simulink library "halout"  (R2021b)
settings: Solver=VariableStepAuto  StartTime=0.0  StopTime=10.0  RelTol=1e-3
undefined symbols (not defined in the file): C_TASK_5MS_S, KHAL_CAN1TxReq_flg, KHAL_CAN2TxReq_flg, KHAL_CAN3TxReq_flg, KHAL_CAN4TxReq_flg, KHAL_CAN5TxReq_flg, KHAL_CAN6TxReq_flg, KHAL_CAN7TxReq_flg, TRUE
libraries: FVT_lib x65, simulink x6
(part 1 of 6)
settings Model: Creator=13168  LastModifiedBy=FVT22063
settings SolverCC: AlgebraicLoopSolver=TrustRegion
settings DataIOCC: SaveFormat=Array  SignalLoggingSaveFormat=ModelDataLogs  ReturnWorkspaceOutputs=off
settings OptimizationCC: BlockReduction=off  BooleanDataType=off
settings DebuggingCC: SaveWithParameterizedLinksMsg=none  UnderspecifiedInitializationDetection=Classic  MergeDetectMultiDrivingBlocksExec=none  SignalResolutionControl=TryResolveAllWithWarning  SFMachineParentedDataDiag=warning
settings HardwareCC: TargetUnknown=on
settings ModelReferenceCC: PropagateSignalLabelsOutOfModel=off
settings ConfigComp: CovMetricSettings=dw  CovSaveCumulativeToWorkspaceVar=on  CovSaveSingleToWorkspaceVar=on

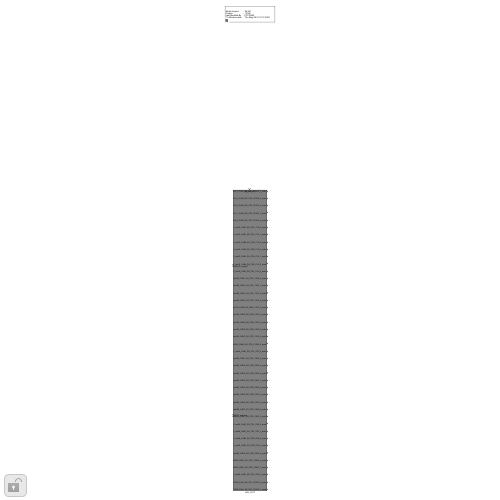
[thumbnail: Simulink's stored preview of the top-level diagram]
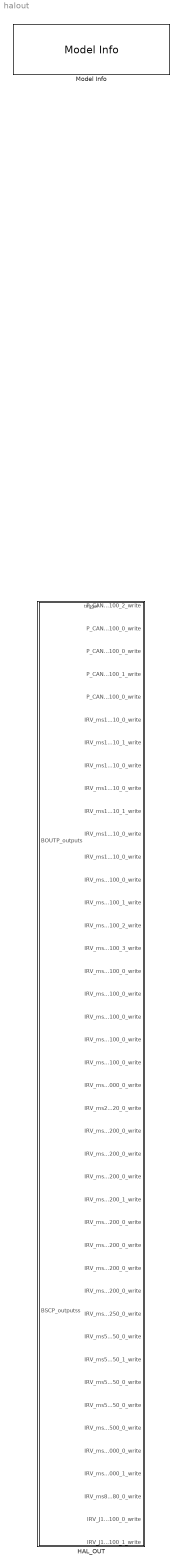
== system halout ==
  HAL_OUT : Subsystem
      settings: RTWSystemCode=Nonreusable function  RTWFcnNameOpts=Use subsystem name  RTWFileNameOpts=Use subsystem name
  Model Info : simulink/Model-Wide Utilities/Model Info  Frame=on  DisplayStringWithTags=|  HorizontalTextAlignment=Left  LeftAlignmentValue=0.02
      | Model Version        : %<ModelVersion>
      | Creator                   : %<Creator>
      | Last Modified By    : %<LastModifiedBy>
      | Modification date    : %<LastModificationDate>

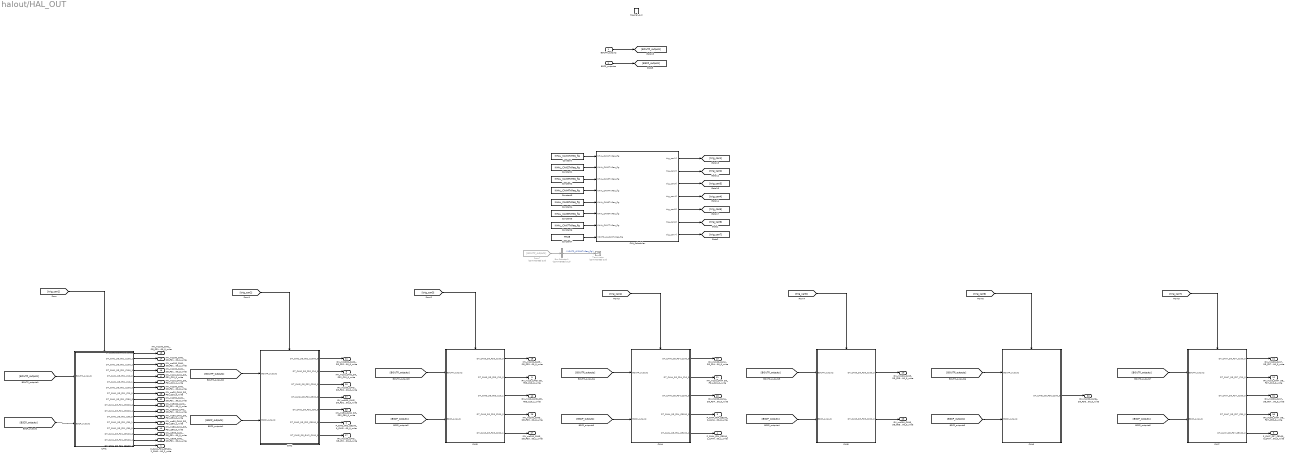
== system halout/HAL_OUT ==
  BOUTP_outputs : Inport  OutDataTypeStr=Bus: BOUTP_outputs
  BSCP_outputss : Inport  Port=2  OutDataTypeStr=Bus: BSCP_outputs
  trig_hal_out : TriggerPort  TriggerType=function-call  VariantControl=(inherit)
  Bus Selector1 : BusSelector  Commented=on  OutputSignals=VOUTP_AllCANTxReq_flg
  CAN1 : Subsystem  TreatAsAtomicUnit=on
  CAN2 : Subsystem  TreatAsAtomicUnit=on
  CAN3 : Subsystem  TreatAsAtomicUnit=on
  CAN4 : Subsystem  TreatAsAtomicUnit=on
  CAN5 : Subsystem  TreatAsAtomicUnit=on
  CAN6 : Subsystem  TreatAsAtomicUnit=on
  CAN7 : Subsystem  TreatAsAtomicUnit=on
  CAN_Scheduler : Stateflow chart  TreatAsAtomicUnit=on
  Constant : Constant  Value=KHAL_CAN1TxReq_flg
  Constant1 : Constant  Value=KHAL_CAN2TxReq_flg
  Constant2 : Constant  Value=KHAL_CAN3TxReq_flg
  Constant3 : Constant  Value=KHAL_CAN4TxReq_flg
  Constant4 : Constant  Value=KHAL_CAN5TxReq_flg
  Constant5 : Constant  Value=KHAL_CAN6TxReq_flg
  Constant6 : Constant  Value=KHAL_CAN7TxReq_flg
  Constant7 : Constant  Value=TRUE
  From7 : From  Commented=on  GotoTag=BOUTP_outputs
  Terminator : Terminator  Commented=on
  P_CAN1_FD1_CE100_2_CAN1_SG_FD1_CE100_2_write : Outport  OutDataTypeStr=Bus: DT_CAN1_SG_FD1_CE100_2
  P_CAN2_FD2_CE100_0_CAN2_SG_FD2_CE100_0_write : Outport  Port=2  OutDataTypeStr=Bus: DT_CAN2_SG_FD2_CE100_0
  P_CAN4_FD4_CE100_0_CAN4_SG_FD4_CE100_0_write : Outport  Port=3  OutDataTypeStr=Bus: DT_CAN4_SG_FD4_CE100_0
  P_CAN4_FD4_CE100_1_CAN4_SG_FD4_CE100_1_write : Outport  Port=4  OutDataTypeStr=Bus: DT_CAN4_SG_FD4_CE100_1
  P_CAN7_FD7_CE100_0_CAN7_SG_FD7_CE100_0_write : Outport  Port=5  OutDataTypeStr=Bus: DT_CAN7_SG_FD7_CE100_0
  IRV_ms10_CAN1_SG_FD1_C10_0_write : Outport  Port=6  OutDataTypeStr=Bus: DT_CAN1_SG_FD1_C10_0
  IRV_ms10_CAN1_SG_FD1_C10_1_write : Outport  Port=7  OutDataTypeStr=Bus: DT_CAN1_SG_FD1_C10_1
  IRV_ms10_CAN2_SG_FD2_C10_0_write : Outport  Port=8  OutDataTypeStr=Bus: DT_CAN2_SG_FD2_C10_0
  IRV_ms10_CAN3_SG_FD3_C10_0_write : Outport  Port=9  OutDataTypeStr=Bus: DT_CAN3_SG_FD3_C10_0
  IRV_ms10_CAN3_SG_FD3_C10_1_write : Outport  Port=10  OutDataTypeStr=Bus: DT_CAN3_SG_FD3_C10_1
  IRV_ms10_CAN4_SG_FD4_C10_0_write : Outport  Port=11  OutDataTypeStr=Bus: DT_CAN4_SG_FD4_C10_0
  IRV_ms10_CAN7_SG_FD7_C10_0_write : Outport  Port=12  OutDataTypeStr=Bus: DT_CAN7_SG_FD7_C10_0
  IRV_ms100_CAN1_SG_FD1_C100_0_write : Outport  Port=13  OutDataTypeStr=Bus: DT_CAN1_SG_FD1_C100_0
  IRV_ms100_CAN1_SG_FD1_C100_1_write : Outport  Port=14  OutDataTypeStr=Bus: DT_CAN1_SG_FD1_C100_1
  IRV_ms100_CAN1_SG_FD1_C100_2_write : Outport  Port=15  OutDataTypeStr=Bus: DT_CAN1_SG_FD1_C100_2
  IRV_ms100_CAN1_SG_FD1_C100_3_write : Outport  Port=16  OutDataTypeStr=Bus: DT_CAN1_SG_FD1_C100_3
  IRV_ms100_CAN2_SG_GW2_C100_0_write : Outport  Port=17  OutDataTypeStr=Bus: DT_CAN2_SG_GW2_C100_0
  IRV_ms100_CAN3_SG_FD3_C100_0_write : Outport  Port=18  OutDataTypeStr=Bus: DT_CAN3_SG_FD3_C100_0
  IRV_ms100_CAN4_SG_FD4_C100_0_write : Outport  Port=19  OutDataTypeStr=Bus: DT_CAN4_SG_FD4_C100_0
  IRV_ms100_CAN5_SG_FD5_C100_0_write : Outport  Port=20  OutDataTypeStr=Bus: DT_CAN5_SG_FD5_C100_0
  IRV_ms100_CAN7_SG_FD7_C100_0_write : Outport  Port=21  OutDataTypeStr=Bus: DT_CAN7_SG_FD7_C100_0
  IRV_ms1000_CAN2_SG_FD2_C1000_0_write : Outport  Port=22  OutDataTypeStr=Bus: DT_CAN2_SG_FD2_C1000_0
  IRV_ms20_CAN1_SG_FD1_C20_0_write : Outport  Port=23  OutDataTypeStr=Bus: DT_CAN1_SG_FD1_C20_0
  IRV_ms200_CAN1_SG_FD1_C200_0_write : Outport  Port=24  OutDataTypeStr=Bus: DT_CAN1_SG_FD1_C200_0
  IRV_ms200_CAN2_SG_FD2_C200_0_write : Outport  Port=25  OutDataTypeStr=Bus: DT_CAN2_SG_FD2_C200_0
  IRV_ms200_CAN3_SG_FD3_C200_0_write : Outport  Port=26  OutDataTypeStr=Bus: DT_CAN3_SG_FD3_C200_0
  IRV_ms200_CAN3_SG_FD3_C200_1_write : Outport  Port=27  OutDataTypeStr=Bus: DT_CAN3_SG_FD3_C200_1
  IRV_ms200_CAN4_SG_FD4_C200_0_write : Outport  Port=28  OutDataTypeStr=Bus: DT_CAN4_SG_FD4_C200_0
  IRV_ms200_CAN5_SG_FD5_C200_0_write : Outport  Port=29  OutDataTypeStr=Bus: DT_CAN5_SG_FD5_C200_0
  IRV_ms200_CAN6_SG_FD6_C200_0_write : Outport  Port=30  OutDataTypeStr=Bus: DT_CAN6_SG_FD6_C200_0
  IRV_ms200_CAN7_SG_FD7_C200_0_write : Outport  Port=31  OutDataTypeStr=Bus: DT_CAN7_SG_FD7_C200_0
  IRV_ms250_CAN1_SG_FD1_C250_0_write : Outport  Port=32  OutDataTypeStr=Bus: DT_CAN1_SG_FD1_C250_0
  IRV_ms50_CAN1_SG_FD1_C50_0_write : Outport  Port=33  OutDataTypeStr=Bus: DT_CAN1_SG_FD1_C50_0
  IRV_ms50_CAN1_SG_FD1_C50_1_write : Outport  Port=34  OutDataTypeStr=Bus: DT_CAN1_SG_FD1_C50_1
  IRV_ms50_CAN2_SG_FD2_C50_0_write : Outport  Port=35  OutDataTypeStr=Bus: DT_CAN2_SG_FD2_C50_0
  IRV_ms50_CAN7_SG_FD7_C50_0_write : Outport  Port=36  OutDataTypeStr=Bus: DT_CAN7_SG_FD7_C50_0
  IRV_ms500_CAN2_SG_FD2_C500_0_write : Outport  Port=37  OutDataTypeStr=Bus: DT_CAN2_SG_FD2_C500_0
  IRV_ms5000_CAN1_SG_FD1_C5000_0_write : Outport  Port=38  OutDataTypeStr=Bus: DT_CAN1_SG_FD1_C5000_0
  IRV_ms5000_CAN1_SG_FD1_C5000_1_write : Outport  Port=39  OutDataTypeStr=Bus: DT_CAN1_SG_FD1_C5000_1
  IRV_ms80_CAN1_SG_FD1_C80_0_write : Outport  Port=40  OutDataTypeStr=Bus: DT_CAN1_SG_FD1_C80_0
  IRV_J1939_CAN1_SG_FD1_CE100_0_write : Outport  Port=41  OutDataTypeStr=Bus: DT_CAN1_SG_FD1_CE100_0
  IRV_J1939_CAN1_SG_FD1_CE100_1_write : Outport  Port=42  OutDataTypeStr=Bus: DT_CAN1_SG_FD1_CE100_1
  wires:
  BSCP_outputss/1 -> [BSCP_outputs]
  BOUTP_outputs/1 -> [BOUTP_outputs]
  Constant1/1 -> CAN_Scheduler/2(KHAL_CAN2TxReq_flg)
  Constant3/1 -> CAN_Scheduler/4(KHAL_CAN4TxReq_flg)
  CAN_Scheduler/1(trig_can1()) -> [trig_can1]
  CAN_Scheduler/2(trig_can2()) -> [trig_can2]
  Constant/1 -> CAN_Scheduler/1(KHAL_CAN1TxReq_flg)
  CAN_Scheduler/4(trig_can4()) -> [trig_can4]
  CAN_Scheduler/5(trig_can5()) -> [trig_can5]
  Constant4/1 -> CAN_Scheduler/5(KHAL_CAN5TxReq_flg)
  Constant2/1 -> CAN_Scheduler/3(KHAL_CAN3TxReq_flg)
  CAN_Scheduler/3(trig_can3()) -> [trig_can3]
  [trig_can1] -> CAN1/Trigger
  [trig_can4] -> CAN4/Trigger
  [trig_can5] -> CAN5/Trigger
  [trig_can2] -> CAN2/Trigger
  Constant5/1 -> CAN_Scheduler/6(KHAL_CAN6TxReq_flg)
  CAN_Scheduler/6(trig_can6()) -> [trig_can6]
  [trig_can6] -> CAN6/Trigger
  [trig_can3] -> CAN3/Trigger
  CAN_Scheduler/7(trig_can7()) -> [trig_can7]
  Constant6/1 -> CAN_Scheduler/7(KHAL_CAN7TxReq_flg)
  [trig_can7] -> CAN7/Trigger
  From7/1 -> Bus Selector1/1
  Bus Selector1/1 -> Terminator/1  "<VOUTP_AllCANTxReq_flg>"
  Constant7/1 -> CAN_Scheduler/8(VOUTP_ALLCANTxReq_flg)
  CAN1/1(DT_CAN1_SG_FD1_C100_0) -> IRV_ms100_CAN1_SG_FD1_C100_0_write/1
  CAN2/2(DT_CAN2_SG_FD2_C10_0) -> IRV_ms10_CAN2_SG_FD2_C10_0_write/1
  CAN7/5(DT_CAN7_SG_FD7_CE100_0) -> P_CAN7_FD7_CE100_0_CAN7_SG_FD7_CE100_0_write/1
  CAN1/2(DT_CAN1_SG_FD1_C100_1) -> IRV_ms100_CAN1_SG_FD1_C100_1_write/1
  [BSCP_outputs] -> CAN2/2(BSCP_outputs)
  [BOUTP_outputs] -> CAN2/1(BOUTP_outputs)
  CAN1/17(DT_CAN1_SG_FD1_CE100_2) -> P_CAN1_FD1_CE100_2_CAN1_SG_FD1_CE100_2_write/1
  [BSCP_outputs] -> CAN1/2(BSCP_outputs)
  CAN7/2(DT_CAN7_SG_FD7_C10_0) -> IRV_ms10_CAN7_SG_FD7_C10_0_write/1
  CAN1/16(DT_CAN1_SG_FD1_CE100_1) -> IRV_J1939_CAN1_SG_FD1_CE100_1_write/1
  CAN2/6(DT_CAN2_SG_FD2_CE100_0) -> P_CAN2_FD2_CE100_0_CAN2_SG_FD2_CE100_0_write/1
  CAN1/15(DT_CAN1_SG_FD1_CE100_0) -> IRV_J1939_CAN1_SG_FD1_CE100_0_write/1
  CAN1/6(DT_CAN1_SG_FD1_C10_1) -> IRV_ms10_CAN1_SG_FD1_C10_1_write/1
  CAN1/14(DT_CAN1_SG_FD1_C80_0) -> IRV_ms80_CAN1_SG_FD1_C80_0_write/1
  CAN1/5(DT_CAN1_SG_FD1_C10_0) -> IRV_ms10_CAN1_SG_FD1_C10_0_write/1
  CAN1/11(DT_CAN1_SG_FD1_C5000_1) -> IRV_ms5000_CAN1_SG_FD1_C5000_1_write/1
  CAN1/10(DT_CAN1_SG_FD1_C5000_0) -> IRV_ms5000_CAN1_SG_FD1_C5000_0_write/1
  CAN2/4(DT_CAN2_SG_FD2_C500_0) -> IRV_ms500_CAN2_SG_FD2_C500_0_write/1
  CAN7/4(DT_CAN7_SG_FD7_C50_0) -> IRV_ms50_CAN7_SG_FD7_C50_0_write/1
  CAN2/5(DT_CAN2_SG_FD2_C50_0) -> IRV_ms50_CAN2_SG_FD2_C50_0_write/1
  CAN1/9(DT_CAN1_SG_FD1_C250_0) -> IRV_ms250_CAN1_SG_FD1_C250_0_write/1
  CAN6/1(DT_CAN6_SG_FD6_C200_0) -> IRV_ms200_CAN6_SG_FD6_C200_0_write/1
  CAN5/2(DT_CAN5_SG_FD5_C200_0) -> IRV_ms200_CAN5_SG_FD5_C200_0_write/1
  CAN4/3(DT_CAN4_SG_FD4_C200_0) -> IRV_ms200_CAN4_SG_FD4_C200_0_write/1
  CAN3/5(DT_CAN3_SG_FD3_C200_1) -> IRV_ms200_CAN3_SG_FD3_C200_1_write/1
  CAN2/3(DT_CAN2_SG_FD2_C200_0) -> IRV_ms200_CAN2_SG_FD2_C200_0_write/1
  CAN1/7(DT_CAN1_SG_FD1_C200_0) -> IRV_ms200_CAN1_SG_FD1_C200_0_write/1
  CAN3/4(DT_CAN3_SG_FD3_C200_0) -> IRV_ms200_CAN3_SG_FD3_C200_0_write/1
  CAN1/8(DT_CAN1_SG_FD1_C20_0) -> IRV_ms20_CAN1_SG_FD1_C20_0_write/1
  CAN3/3(DT_CAN3_SG_FD3_C10_1) -> IRV_ms10_CAN3_SG_FD3_C10_1_write/1
  CAN2/1(DT_CAN2_SG_FD2_C1000_0) -> IRV_ms1000_CAN2_SG_FD2_C1000_0_write/1
  CAN4/4(DT_CAN4_SG_FD4_CE100_0) -> P_CAN4_FD4_CE100_0_CAN4_SG_FD4_CE100_0_write/1
  CAN3/2(DT_CAN3_SG_FD3_C10_0) -> IRV_ms10_CAN3_SG_FD3_C10_0_write/1
  CAN7/1(DT_CAN7_SG_FD7_C100_0) -> IRV_ms100_CAN7_SG_FD7_C100_0_write/1
  CAN1/12(DT_CAN1_SG_FD1_C50_0) -> IRV_ms50_CAN1_SG_FD1_C50_0_write/1
  CAN5/1(DT_CAN5_SG_FD5_C100_0) -> IRV_ms100_CAN5_SG_FD5_C100_0_write/1
  CAN4/1(DT_CAN4_SG_FD4_C100_0) -> IRV_ms100_CAN4_SG_FD4_C100_0_write/1
  CAN3/1(DT_CAN3_SG_FD3_C100_0) -> IRV_ms100_CAN3_SG_FD3_C100_0_write/1
  [BSCP_outputs] -> CAN4/2(BSCP_outputs)
  [BOUTP_outputs] -> CAN3/1(BOUTP_outputs)
  CAN7/3(DT_CAN7_SG_FD7_C200_0) -> IRV_ms200_CAN7_SG_FD7_C200_0_write/1
  [BSCP_outputs] -> CAN3/2(BSCP_outputs)
  CAN4/5(DT_CAN4_SG_FD4_CE100_1) -> P_CAN4_FD4_CE100_1_CAN4_SG_FD4_CE100_1_write/1
  [BOUTP_outputs] -> CAN7/1(BOUTP_outputs)
  [BSCP_outputs] -> CAN7/2(BSCP_outputs)
  [BSCP_outputs] -> CAN6/2(BSCP_outputs)
  CAN1/13(DT_CAN1_SG_FD1_C50_1) -> IRV_ms50_CAN1_SG_FD1_C50_1_write/1
  [BSCP_outputs] -> CAN5/2(BSCP_outputs)
  CAN1/4(DT_CAN1_SG_FD1_C100_3) -> IRV_ms100_CAN1_SG_FD1_C100_3_write/1
  [BOUTP_outputs] -> CAN1/1(BOUTP_outputs)
  [BOUTP_outputs] -> CAN6/1(BOUTP_outputs)
  CAN2/7(DT_CAN2_SG_GW2_C100_0) -> IRV_ms100_CAN2_SG_GW2_C100_0_write/1
  CAN4/2(DT_CAN4_SG_FD4_C10_0) -> IRV_ms10_CAN4_SG_FD4_C10_0_write/1
  CAN1/3(DT_CAN1_SG_FD1_C100_2) -> IRV_ms100_CAN1_SG_FD1_C100_2_write/1
  [BOUTP_outputs] -> CAN5/1(BOUTP_outputs)
  [BOUTP_outputs] -> CAN4/1(BOUTP_outputs)

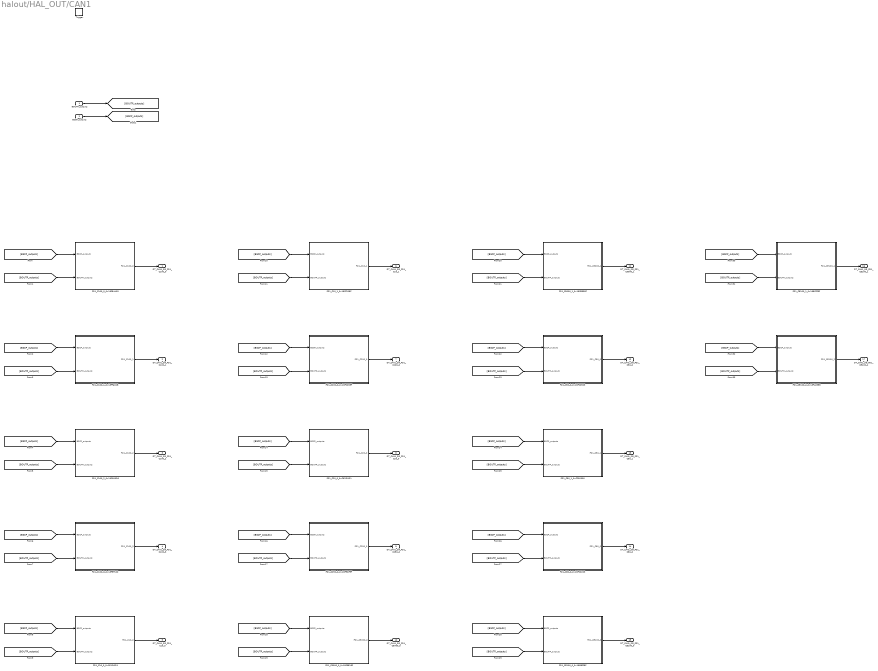
== system halout/HAL_OUT/CAN1 ==
  BOUTP_outputs : Inport  OutDataTypeStr=Bus: BOUTP_outputs
  BSCP_outputs : Inport  Port=2  OutDataTypeStr=Bus: BSCP_outputs
  Trigger : TriggerPort  TriggerType=function-call  VariantControl=(inherit)
  FD1_C100_0_0x18FE4A03 : Subsystem
  FD1_C100_1_0x18FF602B : Subsystem
  FD1_C100_2_0x19F005D0 : Subsystem
  FD1_C100_3_0x18FEF100 : Subsystem
  FD1_C10_0_0xC61D0D1 : Subsystem
  FD1_C10_1_0x18FF20EF : Subsystem
  FD1_C200_0_0x18F003EF : Subsystem
  FD1_C20_0_0xC62D0D1 : Subsystem
  FD1_C250_0_0x18FEDFEF : Subsystem
  FD1_C5000_0_0x18FEE1EF : Subsystem
  FD1_C5000_1_0x18FEE3EF : Subsystem
  FD1_C50_0_0x18F00503 : Subsystem
  FD1_C50_1_0xCF00300 : Subsystem
  FD1_C80_0_0x18F00203 : Subsystem
  FD1_CE100_0_0x18EBFFEF : Subsystem
  FD1_CE100_1_0x18ECFFEF : Subsystem
  FD1_CE100_2_0x18FA05B9 : Subsystem
  DT_CAN1_SG_FD1_C100_0 : Outport  OutDataTypeStr=Bus: DT_CAN1_SG_FD1_C100_0
  DT_CAN1_SG_FD1_C100_1 : Outport  Port=2  OutDataTypeStr=Bus: DT_CAN1_SG_FD1_C100_1
  DT_CAN1_SG_FD1_C100_2 : Outport  Port=3  OutDataTypeStr=Bus: DT_CAN1_SG_FD1_C100_2
  DT_CAN1_SG_FD1_C100_3 : Outport  Port=4  OutDataTypeStr=Bus: DT_CAN1_SG_FD1_C100_3
  DT_CAN1_SG_FD1_C10_0 : Outport  Port=5  OutDataTypeStr=Bus: DT_CAN1_SG_FD1_C10_0
  DT_CAN1_SG_FD1_C10_1 : Outport  Port=6  OutDataTypeStr=Bus: DT_CAN1_SG_FD1_C10_1
  DT_CAN1_SG_FD1_C200_0 : Outport  Port=7  OutDataTypeStr=Bus: DT_CAN1_SG_FD1_C200_0
  DT_CAN1_SG_FD1_C20_0 : Outport  Port=8  OutDataTypeStr=Bus: DT_CAN1_SG_FD1_C20_0
  DT_CAN1_SG_FD1_C250_0 : Outport  Port=9  OutDataTypeStr=Bus: DT_CAN1_SG_FD1_C250_0
  DT_CAN1_SG_FD1_C5000_0 : Outport  Port=10  OutDataTypeStr=Bus: DT_CAN1_SG_FD1_C5000_0
  DT_CAN1_SG_FD1_C5000_1 : Outport  Port=11  OutDataTypeStr=Bus: DT_CAN1_SG_FD1_C5000_1
  DT_CAN1_SG_FD1_C50_0 : Outport  Port=12  OutDataTypeStr=Bus: DT_CAN1_SG_FD1_C50_0
  DT_CAN1_SG_FD1_C50_1 : Outport  Port=13  OutDataTypeStr=Bus: DT_CAN1_SG_FD1_C50_1
  DT_CAN1_SG_FD1_C80_0 : Outport  Port=14  OutDataTypeStr=Bus: DT_CAN1_SG_FD1_C80_0
  DT_CAN1_SG_FD1_CE100_0 : Outport  Port=15  OutDataTypeStr=Bus: DT_CAN1_SG_FD1_CE100_0
  DT_CAN1_SG_FD1_CE100_1 : Outport  Port=16  OutDataTypeStr=Bus: DT_CAN1_SG_FD1_CE100_1
  DT_CAN1_SG_FD1_CE100_2 : Outport  Port=17  OutDataTypeStr=Bus: DT_CAN1_SG_FD1_CE100_2
  wires:
  BOUTP_outputs/1 -> [BOUTP_outputs]
  BSCP_outputs/1 -> [BSCP_outputs]
  [BSCP_outputs] -> FD1_C100_0_0x18FE4A03/1(BSCP_outputs)
  [BOUTP_outputs] -> FD1_C100_0_0x18FE4A03/2(BOUTP_outputs)
  FD1_C100_0_0x18FE4A03/1(FD1_C100_0) -> DT_CAN1_SG_FD1_C100_0/1
  [BSCP_outputs] -> FD1_C100_1_0x18FF602B/1(BSCP_outputs)
  [BOUTP_outputs] -> FD1_C100_1_0x18FF602B/2(BOUTP_outputs)
  FD1_C100_1_0x18FF602B/1(FD1_C100_1) -> DT_CAN1_SG_FD1_C100_1/1
  [BSCP_outputs] -> FD1_C100_2_0x19F005D0/1(BSCP_outputs)
  [BOUTP_outputs] -> FD1_C100_2_0x19F005D0/2(BOUTP_outputs)
  FD1_C100_2_0x19F005D0/1(FD1_C100_2) -> DT_CAN1_SG_FD1_C100_2/1
  [BSCP_outputs] -> FD1_C100_3_0x18FEF100/1(BSCP_outputs)
  [BOUTP_outputs] -> FD1_C100_3_0x18FEF100/2(BOUTP_outputs)
  FD1_C100_3_0x18FEF100/1(FD1_C100_3) -> DT_CAN1_SG_FD1_C100_3/1
  [BSCP_outputs] -> FD1_C10_0_0xC61D0D1/1(BSCP_outputs)
  [BOUTP_outputs] -> FD1_C10_0_0xC61D0D1/2(BOUTP_outputs)
  FD1_C10_0_0xC61D0D1/1(FD1_C10_0) -> DT_CAN1_SG_FD1_C10_0/1
  [BSCP_outputs] -> FD1_C10_1_0x18FF20EF/1(BSCP_outputs)
  [BOUTP_outputs] -> FD1_C10_1_0x18FF20EF/2(BOUTP_outputs)
  FD1_C10_1_0x18FF20EF/1(FD1_C10_1) -> DT_CAN1_SG_FD1_C10_1/1
  [BSCP_outputs] -> FD1_C200_0_0x18F003EF/1(BSCP_outputs)
  [BOUTP_outputs] -> FD1_C200_0_0x18F003EF/2(BOUTP_outputs)
  FD1_C200_0_0x18F003EF/1(FD1_C200_0) -> DT_CAN1_SG_FD1_C200_0/1
  [BSCP_outputs] -> FD1_C20_0_0xC62D0D1/1(BSCP_outputs)
  [BOUTP_outputs] -> FD1_C20_0_0xC62D0D1/2(BOUTP_outputs)
  FD1_C20_0_0xC62D0D1/1(FD1_C20_0) -> DT_CAN1_SG_FD1_C20_0/1
  [BSCP_outputs] -> FD1_C250_0_0x18FEDFEF/1(BSCP_outputs)
  [BOUTP_outputs] -> FD1_C250_0_0x18FEDFEF/2(BOUTP_outputs)
  FD1_C250_0_0x18FEDFEF/1(FD1_C250_0) -> DT_CAN1_SG_FD1_C250_0/1
  [BSCP_outputs] -> FD1_C5000_0_0x18FEE1EF/1(BSCP_outputs)
  [BOUTP_outputs] -> FD1_C5000_0_0x18FEE1EF/2(BOUTP_outputs)
  FD1_C5000_0_0x18FEE1EF/1(FD1_C5000_0) -> DT_CAN1_SG_FD1_C5000_0/1
  [BSCP_outputs] -> FD1_C5000_1_0x18FEE3EF/1(BSCP_outputs)
  [BOUTP_outputs] -> FD1_C5000_1_0x18FEE3EF/2(BOUTP_outputs)
  FD1_C5000_1_0x18FEE3EF/1(FD1_C5000_1) -> DT_CAN1_SG_FD1_C5000_1/1
  [BSCP_outputs] -> FD1_C50_0_0x18F00503/1(BSCP_outputs)
  [BOUTP_outputs] -> FD1_C50_0_0x18F00503/2(BOUTP_outputs)
  FD1_C50_0_0x18F00503/1(FD1_C50_0) -> DT_CAN1_SG_FD1_C50_0/1
  [BSCP_outputs] -> FD1_C50_1_0xCF00300/1(BSCP_outputs)
  [BOUTP_outputs] -> FD1_C50_1_0xCF00300/2(BOUTP_outputs)
  FD1_C50_1_0xCF00300/1(FD1_C50_1) -> DT_CAN1_SG_FD1_C50_1/1
  [BSCP_outputs] -> FD1_C80_0_0x18F00203/1(BSCP_outputs)
  [BOUTP_outputs] -> FD1_C80_0_0x18F00203/2(BOUTP_outputs)
  FD1_C80_0_0x18F00203/1(FD1_C80_0) -> DT_CAN1_SG_FD1_C80_0/1
  [BSCP_outputs] -> FD1_CE100_0_0x18EBFFEF/1(BSCP_outputs)
  [BOUTP_outputs] -> FD1_CE100_0_0x18EBFFEF/2(BOUTP_outputs)
  FD1_CE100_0_0x18EBFFEF/1(FD1_CE100_0) -> DT_CAN1_SG_FD1_CE100_0/1
  [BSCP_outputs] -> FD1_CE100_1_0x18ECFFEF/1(BSCP_outputs)
  [BOUTP_outputs] -> FD1_CE100_1_0x18ECFFEF/2(BOUTP_outputs)
  FD1_CE100_1_0x18ECFFEF/1(FD1_CE100_1) -> DT_CAN1_SG_FD1_CE100_1/1
  [BSCP_outputs] -> FD1_CE100_2_0x18FA05B9/1(BSCP_outputs)
  [BOUTP_outputs] -> FD1_CE100_2_0x18FA05B9/2(BOUTP_outputs)
  FD1_CE100_2_0x18FA05B9/1(FD1_CE100_2) -> DT_CAN1_SG_FD1_CE100_2/1

== system halout/HAL_OUT/CAN2 ==
  BOUTP_outputs : Inport  OutDataTypeStr=Bus: BOUTP_outputs
  BSCP_outputs : Inport  Port=2  OutDataTypeStr=Bus: BSCP_outputs
  Trigger : TriggerPort  TriggerType=function-call  VariantControl=(inherit)
  FD2_C1000_0_0x20E : Subsystem
  FD2_C10_0_0xC61D0D1 : Subsystem
  FD2_C200_0_0x20F : Subsystem
  FD2_C500_0_0x18FA0517 : Subsystem
  FD2_C50_0_0xCFF355A : Subsystem
  FD2_CE100_0_0x209 : Subsystem
  GW2_C100_0_0x20B : Subsystem
  DT_CAN2_SG_FD2_C1000_0 : Outport  OutDataTypeStr=Bus: DT_CAN2_SG_FD2_C1000_0
  DT_CAN2_SG_FD2_C10_0 : Outport  Port=2  OutDataTypeStr=Bus: DT_CAN2_SG_FD2_C10_0
  DT_CAN2_SG_FD2_C200_0 : Outport  Port=3  OutDataTypeStr=Bus: DT_CAN2_SG_FD2_C200_0
  DT_CAN2_SG_FD2_C500_0 : Outport  Port=4  OutDataTypeStr=Bus: DT_CAN2_SG_FD2_C500_0
  DT_CAN2_SG_FD2_C50_0 : Outport  Port=5  OutDataTypeStr=Bus: DT_CAN2_SG_FD2_C50_0
  DT_CAN2_SG_FD2_CE100_0 : Outport  Port=6  OutDataTypeStr=Bus: DT_CAN2_SG_FD2_CE100_0
  DT_CAN2_SG_GW2_C100_0 : Outport  Port=7  OutDataTypeStr=Bus: DT_CAN2_SG_GW2_C100_0
  wires:
  BOUTP_outputs/1 -> [BOUTP_outputs]
  BSCP_outputs/1 -> [BSCP_outputs]
  [BSCP_outputs] -> FD2_C1000_0_0x20E/1(BSCP_outputs)
  [BOUTP_outputs] -> FD2_C1000_0_0x20E/2(BOUTP_outputs)
  FD2_C1000_0_0x20E/1(FD2_C1000_0) -> DT_CAN2_SG_FD2_C1000_0/1
  [BSCP_outputs] -> FD2_C10_0_0xC61D0D1/1(BSCP_outputs)
  [BOUTP_outputs] -> FD2_C10_0_0xC61D0D1/2(BOUTP_outputs)
  FD2_C10_0_0xC61D0D1/1(FD2_C10_0) -> DT_CAN2_SG_FD2_C10_0/1
  [BSCP_outputs] -> FD2_C200_0_0x20F/1(BSCP_outputs)
  [BOUTP_outputs] -> FD2_C200_0_0x20F/2(BOUTP_outputs)
  FD2_C200_0_0x20F/1(FD2_C200_0) -> DT_CAN2_SG_FD2_C200_0/1
  [BSCP_outputs] -> FD2_C500_0_0x18FA0517/1(BSCP_outputs)
  [BOUTP_outputs] -> FD2_C500_0_0x18FA0517/2(BOUTP_outputs)
  FD2_C500_0_0x18FA0517/1(FD2_C500_0) -> DT_CAN2_SG_FD2_C500_0/1
  [BSCP_outputs] -> FD2_C50_0_0xCFF355A/1(BSCP_outputs)
  [BOUTP_outputs] -> FD2_C50_0_0xCFF355A/2(BOUTP_outputs)
  FD2_C50_0_0xCFF355A/1(FD2_C50_0) -> DT_CAN2_SG_FD2_C50_0/1
  [BSCP_outputs] -> FD2_CE100_0_0x209/1(BSCP_outputs)
  [BOUTP_outputs] -> FD2_CE100_0_0x209/2(BOUTP_outputs)
  FD2_CE100_0_0x209/1(FD2_CE100_0) -> DT_CAN2_SG_FD2_CE100_0/1
  [BSCP_outputs] -> GW2_C100_0_0x20B/1(BSCP_outputs)
  [BOUTP_outputs] -> GW2_C100_0_0x20B/2(BOUTP_outputs)
  GW2_C100_0_0x20B/1(GW2_C100_0) -> DT_CAN2_SG_GW2_C100_0/1

== system halout/HAL_OUT/CAN3 ==
  BOUTP_outputs : Inport  OutDataTypeStr=Bus: BOUTP_outputs
  BSCP_outputs : Inport  Port=2  OutDataTypeStr=Bus: BSCP_outputs
  Trigger : TriggerPort  TriggerType=function-call  VariantControl=(inherit)
  Constant : Constant  Value=TRUE
  FD3_C100_0_0x1802F3EF : Subsystem
  FD3_C10_0_0xCF101D0 : Subsystem
  FD3_C10_1_0xCFF05EF : Subsystem
  FD3_C200_0_0x18F003EF : Subsystem
  FD3_C200_1_0x18F001EF : Subsystem
  FD3_VCU2_Tx : Subsystem  mask{CycleTime=10}
      mask prompts: CycleTime "MsgCycleTime_ms"
      mask help: MeasumentTrigerTime
      mask Display: fprintf('Tx Method: Cycle\nMsg Cycletime ms: %3.0f', CycleTime);
  DT_CAN3_SG_FD3_C100_0 : Outport  OutDataTypeStr=Bus: DT_CAN3_SG_FD3_C100_0
  DT_CAN3_SG_FD3_C10_0 : Outport  Port=2  OutDataTypeStr=Bus: DT_CAN3_SG_FD3_C10_0
  DT_CAN3_SG_FD3_C10_1 : Outport  Port=3  OutDataTypeStr=Bus: DT_CAN3_SG_FD3_C10_1
  DT_CAN3_SG_FD3_C200_0 : Outport  Port=4  OutDataTypeStr=Bus: DT_CAN3_SG_FD3_C200_0
  DT_CAN3_SG_FD3_C200_1 : Outport  Port=5  OutDataTypeStr=Bus: DT_CAN3_SG_FD3_C200_1
  wires:
  BOUTP_outputs/1 -> [BOUTP_outputs]
  BSCP_outputs/1 -> [BSCP_outputs]
  [BSCP_outputs] -> FD3_C100_0_0x1802F3EF/1(BSCP_outputs)
  [BOUTP_outputs] -> FD3_C100_0_0x1802F3EF/2(BOUTP_outputs)
  FD3_C100_0_0x1802F3EF/1(FD3_C100_0) -> DT_CAN3_SG_FD3_C100_0/1
  [BSCP_outputs] -> FD3_C10_0_0xCF101D0/1(BSCP_outputs)
  [BOUTP_outputs] -> FD3_C10_0_0xCF101D0/2(BOUTP_outputs)
  FD3_C10_0_0xCF101D0/1(FD3_C10_0) -> DT_CAN3_SG_FD3_C10_0/1
  [BSCP_outputs] -> FD3_C10_1_0xCFF05EF/1(BSCP_outputs)
  [BOUTP_outputs] -> FD3_C10_1_0xCFF05EF/2(BOUTP_outputs)
  FD3_C10_1_0xCFF05EF/1(FD3_C10_1) -> DT_CAN3_SG_FD3_C10_1/1
  [BSCP_outputs] -> FD3_C200_0_0x18F003EF/1(BSCP_outputs)
  [BOUTP_outputs] -> FD3_C200_0_0x18F003EF/2(BOUTP_outputs)
  FD3_C200_0_0x18F003EF/1(FD3_C200_0) -> DT_CAN3_SG_FD3_C200_0/1
  [BSCP_outputs] -> FD3_C200_1_0x18F001EF/1(BSCP_outputs)
  [BOUTP_outputs] -> FD3_C200_1_0x18F001EF/2(BOUTP_outputs)
  FD3_C200_1_0x18F001EF/1(FD3_C200_1) -> DT_CAN3_SG_FD3_C200_1/1
  FD3_VCU2_Tx/1(TxTrigger) -> FD3_C10_1_0xCFF05EF/Trigger
  Constant/1 -> FD3_VCU2_Tx/1(TxReq)

== system halout/HAL_OUT/CAN4 ==
  BOUTP_outputs : Inport  OutDataTypeStr=Bus: BOUTP_outputs
  BSCP_outputs : Inport  Port=2  OutDataTypeStr=Bus: BSCP_outputs
  Trigger : TriggerPort  TriggerType=function-call  VariantControl=(inherit)
  FD4_C100_0_0xCF103D0 : Subsystem
  FD4_C10_0_0xCF101D0 : Subsystem
  FD4_C200_0_0x18F003EF : Subsystem
  FD4_CE100_0_0x209 : Subsystem
  FD4_CE100_1_0x210 : Subsystem
  DT_CAN4_SG_FD4_C100_0 : Outport  OutDataTypeStr=Bus: DT_CAN4_SG_FD4_C100_0
  DT_CAN4_SG_FD4_C10_0 : Outport  Port=2  OutDataTypeStr=Bus: DT_CAN4_SG_FD4_C10_0
  DT_CAN4_SG_FD4_C200_0 : Outport  Port=3  OutDataTypeStr=Bus: DT_CAN4_SG_FD4_C200_0
  DT_CAN4_SG_FD4_CE100_0 : Outport  Port=4  OutDataTypeStr=Bus: DT_CAN4_SG_FD4_CE100_0
  DT_CAN4_SG_FD4_CE100_1 : Outport  Port=5  OutDataTypeStr=Bus: DT_CAN4_SG_FD4_CE100_1
  wires:
  BOUTP_outputs/1 -> [BOUTP_outputs]
  BSCP_outputs/1 -> [BSCP_outputs]
  [BSCP_outputs] -> FD4_C100_0_0xCF103D0/1(BSCP_outputs)
  [BOUTP_outputs] -> FD4_C100_0_0xCF103D0/2(BOUTP_outputs)
  FD4_C100_0_0xCF103D0/1(FD4_C100_0) -> DT_CAN4_SG_FD4_C100_0/1
  [BSCP_outputs] -> FD4_C10_0_0xCF101D0/1(BSCP_outputs)
  [BOUTP_outputs] -> FD4_C10_0_0xCF101D0/2(BOUTP_outputs)
  FD4_C10_0_0xCF101D0/1(FD4_C10_0) -> DT_CAN4_SG_FD4_C10_0/1
  [BSCP_outputs] -> FD4_C200_0_0x18F003EF/1(BSCP_outputs)
  [BOUTP_outputs] -> FD4_C200_0_0x18F003EF/2(BOUTP_outputs)
  FD4_C200_0_0x18F003EF/1(FD4_C200_0) -> DT_CAN4_SG_FD4_C200_0/1
  [BSCP_outputs] -> FD4_CE100_0_0x209/1(BSCP_outputs)
  [BOUTP_outputs] -> FD4_CE100_0_0x209/2(BOUTP_outputs)
  FD4_CE100_0_0x209/1(FD4_CE100_0) -> DT_CAN4_SG_FD4_CE100_0/1
  [BSCP_outputs] -> FD4_CE100_1_0x210/1(BSCP_outputs)
  [BOUTP_outputs] -> FD4_CE100_1_0x210/2(BOUTP_outputs)
  FD4_CE100_1_0x210/1(FD4_CE100_1) -> DT_CAN4_SG_FD4_CE100_1/1

== system halout/HAL_OUT/CAN5 ==
  BOUTP_outputs : Inport  OutDataTypeStr=Bus: BOUTP_outputs
  BSCP_outputs : Inport  Port=2  OutDataTypeStr=Bus: BSCP_outputs
  Trigger : TriggerPort  TriggerType=function-call  VariantControl=(inherit)
  FD5_C100_0_0x18F348D0 : Subsystem
  FD5_C200_0_0x20D : Subsystem
  DT_CAN5_SG_FD5_C100_0 : Outport  OutDataTypeStr=Bus: DT_CAN5_SG_FD5_C100_0
  DT_CAN5_SG_FD5_C200_0 : Outport  Port=2  OutDataTypeStr=Bus: DT_CAN5_SG_FD5_C200_0
  wires:
  BOUTP_outputs/1 -> [BOUTP_outputs]
  BSCP_outputs/1 -> [BSCP_outputs]
  [BSCP_outputs] -> FD5_C100_0_0x18F348D0/1(BSCP_outputs)
  [BOUTP_outputs] -> FD5_C100_0_0x18F348D0/2(BOUTP_outputs)
  FD5_C100_0_0x18F348D0/1(FD5_C100_0) -> DT_CAN5_SG_FD5_C100_0/1
  [BSCP_outputs] -> FD5_C200_0_0x20D/1(BSCP_outputs)
  [BOUTP_outputs] -> FD5_C200_0_0x20D/2(BOUTP_outputs)
  FD5_C200_0_0x20D/1(FD5_C200_0) -> DT_CAN5_SG_FD5_C200_0/1

== system halout/HAL_OUT/CAN6 ==
  BOUTP_outputs : Inport  OutDataTypeStr=Bus: BOUTP_outputs
  BSCP_outputs : Inport  Port=2  OutDataTypeStr=Bus: BSCP_outputs
  Trigger : TriggerPort  TriggerType=function-call  VariantControl=(inherit)
  FD6_C200_0_0x20C : Subsystem
  DT_CAN6_SG_FD6_C200_0 : Outport  OutDataTypeStr=Bus: DT_CAN6_SG_FD6_C200_0
  wires:
  BOUTP_outputs/1 -> [BOUTP_outputs]
  BSCP_outputs/1 -> [BSCP_outputs]
  [BSCP_outputs] -> FD6_C200_0_0x20C/1(BSCP_outputs)
  [BOUTP_outputs] -> FD6_C200_0_0x20C/2(BOUTP_outputs)
  FD6_C200_0_0x20C/1(FD6_C200_0) -> DT_CAN6_SG_FD6_C200_0/1

== system halout/HAL_OUT/CAN7 ==
  BOUTP_outputs : Inport  OutDataTypeStr=Bus: BOUTP_outputs
  BSCP_outputs : Inport  Port=2  OutDataTypeStr=Bus: BSCP_outputs
  Trigger : TriggerPort  TriggerType=function-call  VariantControl=(inherit)
  FD7_C100_0_0x19F005D0 : Subsystem
  FD7_C10_0_0xC61D0D1 : Subsystem
  FD7_C200_0_0x18F003EF : Subsystem
  FD7_C50_0_0xCF00300 : Subsystem
  FD7_CE100_0_0x18FA05B9 : Subsystem
  DT_CAN7_SG_FD7_C100_0 : Outport  OutDataTypeStr=Bus: DT_CAN7_SG_FD7_C100_0
  DT_CAN7_SG_FD7_C10_0 : Outport  Port=2  OutDataTypeStr=Bus: DT_CAN7_SG_FD7_C10_0
  DT_CAN7_SG_FD7_C200_0 : Outport  Port=3  OutDataTypeStr=Bus: DT_CAN7_SG_FD7_C200_0
  DT_CAN7_SG_FD7_C50_0 : Outport  Port=4  OutDataTypeStr=Bus: DT_CAN7_SG_FD7_C50_0
  DT_CAN7_SG_FD7_CE100_0 : Outport  Port=5  OutDataTypeStr=Bus: DT_CAN7_SG_FD7_CE100_0
  wires:
  BOUTP_outputs/1 -> [BOUTP_outputs]
  BSCP_outputs/1 -> [BSCP_outputs]
  [BSCP_outputs] -> FD7_C100_0_0x19F005D0/1(BSCP_outputs)
  [BOUTP_outputs] -> FD7_C100_0_0x19F005D0/2(BOUTP_outputs)
  FD7_C100_0_0x19F005D0/1(FD7_C100_0) -> DT_CAN7_SG_FD7_C100_0/1
  [BSCP_outputs] -> FD7_C10_0_0xC61D0D1/1(BSCP_outputs)
  [BOUTP_outputs] -> FD7_C10_0_0xC61D0D1/2(BOUTP_outputs)
  FD7_C10_0_0xC61D0D1/1(FD7_C10_0) -> DT_CAN7_SG_FD7_C10_0/1
  [BSCP_outputs] -> FD7_C200_0_0x18F003EF/1(BSCP_outputs)
  [BOUTP_outputs] -> FD7_C200_0_0x18F003EF/2(BOUTP_outputs)
  FD7_C200_0_0x18F003EF/1(FD7_C200_0) -> DT_CAN7_SG_FD7_C200_0/1
  [BSCP_outputs] -> FD7_C50_0_0xCF00300/1(BSCP_outputs)
  [BOUTP_outputs] -> FD7_C50_0_0xCF00300/2(BOUTP_outputs)
  FD7_C50_0_0xCF00300/1(FD7_C50_0) -> DT_CAN7_SG_FD7_C50_0/1
  [BSCP_outputs] -> FD7_CE100_0_0x18FA05B9/1(BSCP_outputs)
  [BOUTP_outputs] -> FD7_CE100_0_0x18FA05B9/2(BOUTP_outputs)
  FD7_CE100_0_0x18FA05B9/1(FD7_CE100_0) -> DT_CAN7_SG_FD7_CE100_0/1

== system halout/HAL_OUT/CAN1/FD1_C100_0_0x18FE4A03 ==
  BSCP_outputs : Inport  OutDataTypeStr=Bus: BSCP_outputs
  BOUTP_outputs : Inport  Port=2  OutDataTypeStr=Bus: BOUTP_outputs
  VCUEBSRd4BR : Subsystem
  bus_creator : BusCreator  Inputs=1  OutDataTypeStr=Bus: DT_CAN1_SG_FD1_C100_0  NonVirtualBus=on
  bus_selector : BusSelector  OutputSignals=VOUTP_VCUEBSRd4BR_enum
  FD1_C100_0 : Outport
  wires:
  BSCP_outputs/1 -> [BSCP_outputs]
  BOUTP_outputs/1 -> [BOUTP_outputs]
  [CAN1_VCUEBSRd4BR] -> bus_creator/1  "CAN1_VCUEBSRd4BR"
  bus_creator/1 -> FD1_C100_0/1
  VCUEBSRd4BR/1(CAN1_VCUEBSRd4BR) -> [CAN1_VCUEBSRd4BR]
  bus_selector/1 -> VCUEBSRd4BR/1(VCUEBSRd4BR)  "<VOUTP_VCUEBSRd4BR_enum>"
  [BOUTP_outputs] -> bus_selector/1

== system halout/HAL_OUT/CAN1/FD1_C100_1_0x18FF602B ==
  BSCP_outputs : Inport  OutDataTypeStr=Bus: BSCP_outputs
  BOUTP_outputs : Inport  Port=2  OutDataTypeStr=Bus: BOUTP_outputs
  VCUEBSHBSw : Subsystem
  VCUEBSHHSw : Subsystem
  bus_creator : BusCreator  Inputs=2  OutDataTypeStr=Bus: DT_CAN1_SG_FD1_C100_1  NonVirtualBus=on
  bus_selector : BusSelector  OutputSignals=VOUTP_VCUEBSHBSw_enum
  bus_selector1 : BusSelector  OutputSignals=VOUTP_VCUEBSHHSw_enum
  FD1_C100_1 : Outport
  wires:
  BSCP_outputs/1 -> [BSCP_outputs]
  BOUTP_outputs/1 -> [BOUTP_outputs]
  [CAN1_VCUEBSHBSw] -> bus_creator/1  "CAN1_VCUEBSHBSw"
  [CAN1_VCUEBSHHSw] -> bus_creator/2  "CAN1_VCUEBSHHSw"
  bus_creator/1 -> FD1_C100_1/1
  VCUEBSHBSw/1(CAN1_VCUEBSHBSw) -> [CAN1_VCUEBSHBSw]
  VCUEBSHHSw/1(CAN1_VCUEBSHHSw) -> [CAN1_VCUEBSHHSw]
  bus_selector/1 -> VCUEBSHBSw/1(VCUEBSHBSw)  "<VOUTP_VCUEBSHBSw_enum>"
  [BOUTP_outputs] -> bus_selector/1
  bus_selector1/1 -> VCUEBSHHSw/1(VCUEBSHHSw)  "<VOUTP_VCUEBSHHSw_enum>"
  [BOUTP_outputs] -> bus_selector1/1

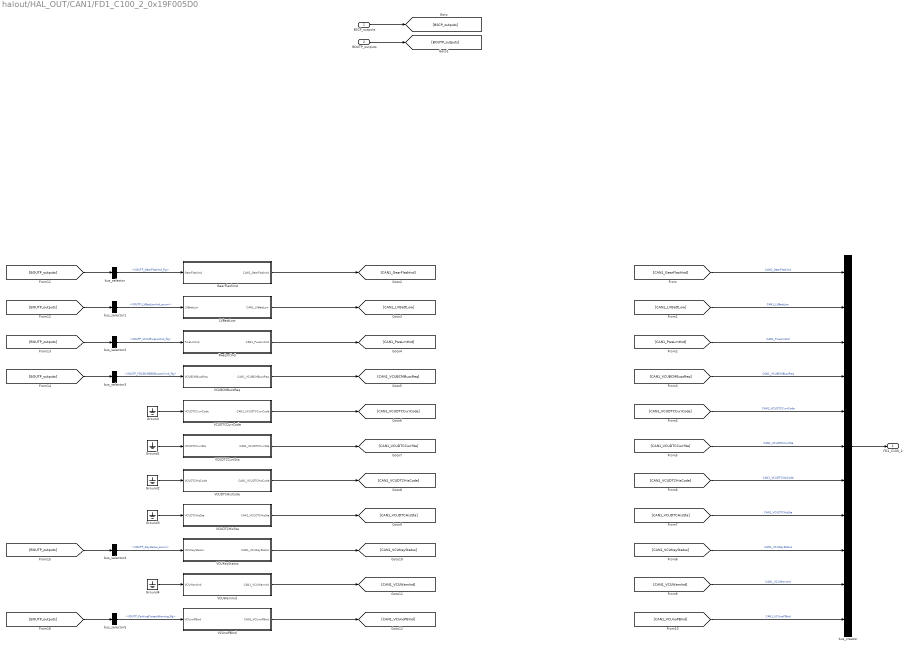
== system halout/HAL_OUT/CAN1/FD1_C100_2_0x19F005D0 ==
  BSCP_outputs : Inport  OutDataTypeStr=Bus: BSCP_outputs
  BOUTP_outputs : Inport  Port=2  OutDataTypeStr=Bus: BOUTP_outputs
  GearFlashInd : Subsystem
  Ground{,1..4} (5 alike) : Ground
  LVBattLow : Subsystem
  PweLmtInd : Subsystem
  VCUBCMBuzzReq : Subsystem
  VCUDTCCurrCode : Subsystem
  VCUDTCCurrSta : Subsystem
  VCUDTCHisCode : Subsystem
  VCUDTCHisSta : Subsystem
  VCUKeyStatus : Subsystem
  VCUWarnInd : Subsystem
  VCUnoPBInd : Subsystem
  bus_creator : BusCreator  Inputs=11  OutDataTypeStr=Bus: DT_CAN1_SG_FD1_C100_2  NonVirtualBus=on
  bus_selector : BusSelector  OutputSignals=VOUTP_GearFlashInd_flg
  bus_selector1 : BusSelector  OutputSignals=VOUTP_LVBattLowInd_enum
  bus_selector2 : BusSelector  OutputSignals=VOUTP_VCU4PweLmtInd_flg
  bus_selector3 : BusSelector  OutputSignals=VOUTP_FDCBCMBSDBuzzerCmd_flg
  bus_selector4 : BusSelector  OutputSignals=VOUTP_Keystatus_enum
  bus_selector5 : BusSelector  OutputSignals=VOUTP_ParkingProtectWarning_flg
  FD1_C100_2 : Outport
  wires:
  BSCP_outputs/1 -> [BSCP_outputs]
  BOUTP_outputs/1 -> [BOUTP_outputs]
  [CAN1_GearFlashInd] -> bus_creator/1  "CAN1_GearFlashInd"
  [CAN1_LVBattLow] -> bus_creator/2  "CAN1_LVBattLow"
  [CAN1_PweLmtInd] -> bus_creator/3  "CAN1_PweLmtInd"
  [CAN1_VCUBCMBuzzReq] -> bus_creator/4  "CAN1_VCUBCMBuzzReq"
  [CAN1_VCUDTCCurrCode] -> bus_creator/5  "CAN1_VCUDTCCurrCode"
  [CAN1_VCUDTCCurrSta] -> bus_creator/6  "CAN1_VCUDTCCurrSta"
  [CAN1_VCUDTCHisCode] -> bus_creator/7  "CAN1_VCUDTCHisCode"
  [CAN1_VCUDTCHisSta] -> bus_creator/8  "CAN1_VCUDTCHisSta"
  [CAN1_VCUKeyStatus] -> bus_creator/9  "CAN1_VCUKeyStatus"
  [CAN1_VCUWarnInd] -> bus_creator/10  "CAN1_VCUWarnInd"
  [CAN1_VCUnoPBInd] -> bus_creator/11  "CAN1_VCUnoPBInd"
  bus_creator/1 -> FD1_C100_2/1
  GearFlashInd/1(CAN1_GearFlashInd) -> [CAN1_GearFlashInd]
  LVBattLow/1(CAN1_LVBattLow) -> [CAN1_LVBattLow]
  PweLmtInd/1(CAN1_PweLmtInd) -> [CAN1_PweLmtInd]
  VCUBCMBuzzReq/1(CAN1_VCUBCMBuzzReq) -> [CAN1_VCUBCMBuzzReq]
  VCUDTCCurrCode/1(CAN1_VCUDTCCurrCode) -> [CAN1_VCUDTCCurrCode]
  VCUDTCCurrSta/1(CAN1_VCUDTCCurrSta) -> [CAN1_VCUDTCCurrSta]
  VCUDTCHisCode/1(CAN1_VCUDTCHisCode) -> [CAN1_VCUDTCHisCode]
  VCUDTCHisSta/1(CAN1_VCUDTCHisSta) -> [CAN1_VCUDTCHisSta]
  VCUKeyStatus/1(CAN1_VCUKeyStatus) -> [CAN1_VCUKeyStatus]
  VCUWarnInd/1(CAN1_VCUWarnInd) -> [CAN1_VCUWarnInd]
  VCUnoPBInd/1(CAN1_VCUnoPBInd) -> [CAN1_VCUnoPBInd]
  bus_selector/1 -> GearFlashInd/1(GearFlashInd)  "<VOUTP_GearFlashInd_flg>"
  [BOUTP_outputs] -> bus_selector/1
  bus_selector1/1 -> LVBattLow/1(LVBattLow)  "<VOUTP_LVBattLowInd_enum>"
  [BOUTP_outputs] -> bus_selector1/1
  bus_selector2/1 -> PweLmtInd/1(PweLmtInd)  "<VOUTP_VCU4PweLmtInd_flg>"
  [BOUTP_outputs] -> bus_selector2/1
  bus_selector3/1 -> VCUBCMBuzzReq/1(VCUBCMBuzzReq)  "<VOUTP_FDCBCMBSDBuzzerCmd_flg>"
  [BOUTP_outputs] -> bus_selector3/1
  Ground/1 -> VCUDTCCurrCode/1(VCUDTCCurrCode)
  Ground1/1 -> VCUDTCCurrSta/1(VCUDTCCurrSta)
  Ground2/1 -> VCUDTCHisCode/1(VCUDTCHisCode)
  Ground3/1 -> VCUDTCHisSta/1(VCUDTCHisSta)
  bus_selector4/1 -> VCUKeyStatus/1(VCUKeyStatus)  "<VOUTP_Keystatus_enum>"
  [BOUTP_outputs] -> bus_selector4/1
  Ground4/1 -> VCUWarnInd/1(VCUWarnInd)
  bus_selector5/1 -> VCUnoPBInd/1(VCUnoPBInd)  "<VOUTP_ParkingProtectWarning_flg>"
  [BOUTP_outputs] -> bus_selector5/1

== system halout/HAL_OUT/CAN1/FD1_C100_3_0x18FEF100 ==
  BSCP_outputs : Inport  OutDataTypeStr=Bus: BSCP_outputs
  BOUTP_outputs : Inport  Port=2  OutDataTypeStr=Bus: BOUTP_outputs
  BrakeSW : Subsystem
  Ground : Ground
  Ground1 : Ground
  VCUVehSpd : Subsystem
  bus_creator : BusCreator  Inputs=2  OutDataTypeStr=Bus: DT_CAN1_SG_FD1_C100_3  NonVirtualBus=on
  FD1_C100_3 : Outport
  wires:
  BSCP_outputs/1 -> [BSCP_outputs]
  BOUTP_outputs/1 -> [BOUTP_outputs]
  [CAN1_BrakeSW] -> bus_creator/1  "CAN1_BrakeSW"
  [CAN1_VCUVehSpd] -> bus_creator/2  "CAN1_VCUVehSpd"
  bus_creator/1 -> FD1_C100_3/1
  BrakeSW/1(CAN1_BrakeSW) -> [CAN1_BrakeSW]
  VCUVehSpd/1(CAN1_VCUVehSpd) -> [CAN1_VCUVehSpd]
  Ground/1 -> BrakeSW/1(BrakeSW)
  Ground1/1 -> VCUVehSpd/1(VCUVehSpd)

== system halout/HAL_OUT/CAN1/FD1_C10_0_0xC61D0D1 ==
  BSCP_outputs : Inport  OutDataTypeStr=Bus: BSCP_outputs
  BOUTP_outputs : Inport  Port=2  OutDataTypeStr=Bus: BOUTP_outputs
  VehActDriveDirect : Subsystem
  bus_creator : BusCreator  Inputs=1  OutDataTypeStr=Bus: DT_CAN1_SG_FD1_C10_0  NonVirtualBus=on
  bus_selector : BusSelector  OutputSignals=VOUTP_EVCU1ActDrvMode_enum
  FD1_C10_0 : Outport
  wires:
  BSCP_outputs/1 -> [BSCP_outputs]
  BOUTP_outputs/1 -> [BOUTP_outputs]
  [CAN1_VehActDriveDirect] -> bus_creator/1  "CAN1_VehActDriveDirect"
  bus_creator/1 -> FD1_C10_0/1
  VehActDriveDirect/1(CAN1_VehActDriveDirect) -> [CAN1_VehActDriveDirect]
  bus_selector/1 -> VehActDriveDirect/1(VehActDriveDirect)  "<VOUTP_EVCU1ActDrvMode_enum>"
  [BOUTP_outputs] -> bus_selector/1

== system halout/HAL_OUT/CAN1/FD1_C10_1_0x18FF20EF ==
  BSCP_outputs : Inport  OutDataTypeStr=Bus: BSCP_outputs
  BOUTP_outputs : Inport  Port=2  OutDataTypeStr=Bus: BOUTP_outputs
  ActEMOutSftSpd : Subsystem
  ActEMpTrq : Subsystem
  ActEMpTrqHrls : Subsystem
  ActMaxAvaEMRecpTrq : Subsystem
  DrvDemEMRtapTrq : Subsystem
  EMTrqModeDrvBrk : Subsystem
  RetSelNonEng : Subsystem
  SACtrlDev : Subsystem
  bus_creator : BusCreator  Inputs=8  OutDataTypeStr=Bus: DT_CAN1_SG_FD1_C10_1  NonVirtualBus=on
  bus_selector : BusSelector  OutputSignals=VOUTP_EMRC1ActEMOutSftSpd_rpm
  bus_selector1 : BusSelector  OutputSignals=VOUTP_EMRC1ActEMpTrq_pct
  bus_selector2 : BusSelector  OutputSignals=VOUTP_EMRC1ActEMpTrqHrls_pct
  bus_selector3 : BusSelector  OutputSignals=VOUTP_EMRC1ActMaxAvaEMRecpTrq_pct
  bus_selector4 : BusSelector  OutputSignals=VOUTP_EMRC1DrvDemEMRtapTrq_pct
  bus_selector5 : BusSelector  OutputSignals=VOUTP_EMRC1EMTquModeDrvBrk_enum
  bus_selector6 : BusSelector  OutputSignals=VOUTP_EMRC1RetSelNonEng_pct
  bus_selector7 : BusSelector  OutputSignals=VOUTP_EMRC1SACtrlDev_cnt
  FD1_C10_1 : Outport
  wires:
  BSCP_outputs/1 -> [BSCP_outputs]
  BOUTP_outputs/1 -> [BOUTP_outputs]
  [CAN1_ActEMOutSftSpd] -> bus_creator/1  "CAN1_ActEMOutSftSpd"
  [CAN1_ActEMpTrq] -> bus_creator/2  "CAN1_ActEMpTrq"
  [CAN1_ActEMpTrqHrls] -> bus_creator/3  "CAN1_ActEMpTrqHrls"
  [CAN1_ActMaxAvaEMRecpTrq] -> bus_creator/4  "CAN1_ActMaxAvaEMRecpTrq"
  [CAN1_DrvDemEMRtapTrq] -> bus_creator/5  "CAN1_DrvDemEMRtapTrq"
  [CAN1_EMTrqModeDrvBrk] -> bus_creator/6  "CAN1_EMTrqModeDrvBrk"
  [CAN1_RetSelNonEng] -> bus_creator/7  "CAN1_RetSelNonEng"
  [CAN1_SACtrlDev] -> bus_creator/8  "CAN1_SACtrlDev"
  bus_creator/1 -> FD1_C10_1/1
  ActEMOutSftSpd/1(CAN1_ActEMOutSftSpd) -> [CAN1_ActEMOutSftSpd]
  ActEMpTrq/1(CAN1_ActEMpTrq) -> [CAN1_ActEMpTrq]
  ActEMpTrqHrls/1(CAN1_ActEMpTrqHrls) -> [CAN1_ActEMpTrqHrls]
  ActMaxAvaEMRecpTrq/1(CAN1_ActMaxAvaEMRecpTrq) -> [CAN1_ActMaxAvaEMRecpTrq]
  DrvDemEMRtapTrq/1(CAN1_DrvDemEMRtapTrq) -> [CAN1_DrvDemEMRtapTrq]
  EMTrqModeDrvBrk/1(CAN1_EMTrqModeDrvBrk) -> [CAN1_EMTrqModeDrvBrk]
  RetSelNonEng/1(CAN1_RetSelNonEng) -> [CAN1_RetSelNonEng]
  SACtrlDev/1(CAN1_SACtrlDev) -> [CAN1_SACtrlDev]
  bus_selector/1 -> ActEMOutSftSpd/1(ActEMOutSftSpd)  "<VOUTP_EMRC1ActEMOutSftSpd_rpm>"
  [BOUTP_outputs] -> bus_selector/1
  bus_selector1/1 -> ActEMpTrq/1(ActEMpTrq)  "<VOUTP_EMRC1ActEMpTrq_pct>"
  [BOUTP_outputs] -> bus_selector1/1
  bus_selector2/1 -> ActEMpTrqHrls/1(ActEMpTrqHrls)  "<VOUTP_EMRC1ActEMpTrqHrls_pct>"
  [BOUTP_outputs] -> bus_selector2/1
  bus_selector3/1 -> ActMaxAvaEMRecpTrq/1(ActMaxAvaEMRecpTrq)  "<VOUTP_EMRC1ActMaxAvaEMRecpTrq_pct>"
  [BOUTP_outputs] -> bus_selector3/1
  bus_selector4/1 -> DrvDemEMRtapTrq/1(DrvDemEMRtapTrq)  "<VOUTP_EMRC1DrvDemEMRtapTrq_pct>"
  [BOUTP_outputs] -> bus_selector4/1
  bus_selector5/1 -> EMTrqModeDrvBrk/1(EMTrqModeDrvBrk)  "<VOUTP_EMRC1EMTquModeDrvBrk_enum>"
  [BOUTP_outputs] -> bus_selector5/1
  bus_selector6/1 -> RetSelNonEng/1(RetSelNonEng)  "<VOUTP_EMRC1RetSelNonEng_pct>"
  [BOUTP_outputs] -> bus_selector6/1
  bus_selector7/1 -> SACtrlDev/1(SACtrlDev)  "<VOUTP_EMRC1SACtrlDev_cnt>"
  [BOUTP_outputs] -> bus_selector7/1

== system halout/HAL_OUT/CAN1/FD1_C200_0_0x18F003EF ==
  BSCP_outputs : Inport  OutDataTypeStr=Bus: BSCP_outputs
  BOUTP_outputs : Inport  Port=2  OutDataTypeStr=Bus: BOUTP_outputs
  SysPowerMode : Subsystem
  bus_creator : BusCreator  Inputs=1  OutDataTypeStr=Bus: DT_CAN1_SG_FD1_C200_0  NonVirtualBus=on
  bus_selector : BusSelector  OutputSignals=VOUTP_SysPowerMode_enum
  FD1_C200_0 : Outport
  wires:
  BSCP_outputs/1 -> [BSCP_outputs]
  BOUTP_outputs/1 -> [BOUTP_outputs]
  [CAN1_SysPowerMode] -> bus_creator/1  "CAN1_SysPowerMode"
  bus_creator/1 -> FD1_C200_0/1
  SysPowerMode/1(CAN1_SysPowerMode) -> [CAN1_SysPowerMode]
  bus_selector/1 -> SysPowerMode/1(SysPowerMode)  "<VOUTP_SysPowerMode_enum>"
  [BOUTP_outputs] -> bus_selector/1

== system halout/HAL_OUT/CAN1/FD1_C20_0_0xC62D0D1 ==
  BSCP_outputs : Inport  OutDataTypeStr=Bus: BSCP_outputs
  BOUTP_outputs : Inport  Port=2  OutDataTypeStr=Bus: BOUTP_outputs
  DCCurr : Subsystem
  DCVol : Subsystem
  MaxTorqAvail : Subsystem
  MinTorqAvail : Subsystem
  bus_creator : BusCreator  Inputs=4  OutDataTypeStr=Bus: DT_CAN1_SG_FD1_C20_0  NonVirtualBus=on
  bus_selector : BusSelector  OutputSignals=VOUTP_DCCurr_A
  bus_selector1 : BusSelector  OutputSignals=VOUTP_DCVol_V
  bus_selector2 : BusSelector  OutputSignals=VOUTP_EVCU2MaxTorqAvail_pct
  bus_selector3 : BusSelector  OutputSignals=VOUTP_EVCU2MinTorqAvail_pct
  FD1_C20_0 : Outport
  wires:
  BSCP_outputs/1 -> [BSCP_outputs]
  BOUTP_outputs/1 -> [BOUTP_outputs]
  [CAN1_DCCurr] -> bus_creator/1  "CAN1_DCCurr"
  [CAN1_DCVol] -> bus_creator/2  "CAN1_DCVol"
  [CAN1_MaxTorqAvail] -> bus_creator/3  "CAN1_MaxTorqAvail"
  [CAN1_MinTorqAvail] -> bus_creator/4  "CAN1_MinTorqAvail"
  bus_creator/1 -> FD1_C20_0/1
  DCCurr/1(CAN1_DCCurr) -> [CAN1_DCCurr]
  DCVol/1(CAN1_DCVol) -> [CAN1_DCVol]
  MaxTorqAvail/1(CAN1_MaxTorqAvail) -> [CAN1_MaxTorqAvail]
  MinTorqAvail/1(CAN1_MinTorqAvail) -> [CAN1_MinTorqAvail]
  bus_selector/1 -> DCCurr/1(DCCurr)  "<VOUTP_DCCurr_A>"
  [BOUTP_outputs] -> bus_selector/1
  bus_selector1/1 -> DCVol/1(DCVol)  "<VOUTP_DCVol_V>"
  [BOUTP_outputs] -> bus_selector1/1
  bus_selector2/1 -> MaxTorqAvail/1(MaxTorqAvail)  "<VOUTP_EVCU2MaxTorqAvail_pct>"
  [BOUTP_outputs] -> bus_selector2/1
  bus_selector3/1 -> MinTorqAvail/1(MinTorqAvail)  "<VOUTP_EVCU2MinTorqAvail_pct>"
  [BOUTP_outputs] -> bus_selector3/1

== system halout/HAL_OUT/CAN1/FD1_C250_0_0x18FEDFEF ==
  BSCP_outputs : Inport  OutDataTypeStr=Bus: BSCP_outputs
  BOUTP_outputs : Inport  Port=2  OutDataTypeStr=Bus: BOUTP_outputs
  EMParasLoss : Subsystem
  NFricPercTorq : Subsystem
  bus_creator : BusCreator  Inputs=2  OutDataTypeStr=Bus: DT_CAN1_SG_FD1_C250_0  NonVirtualBus=on
  bus_selector : BusSelector  OutputSignals=VOUTP_EEC3EMPressLoss_pct
  bus_selector1 : BusSelector  OutputSignals=VOUTP_EEC3NFricPercTorq_pct
  FD1_C250_0 : Outport
  wires:
  BSCP_outputs/1 -> [BSCP_outputs]
  BOUTP_outputs/1 -> [BOUTP_outputs]
  [CAN1_EMParasLoss] -> bus_creator/1  "CAN1_EMParasLoss"
  [CAN1_NFricPercTorq] -> bus_creator/2  "CAN1_NFricPercTorq"
  bus_creator/1 -> FD1_C250_0/1
  EMParasLoss/1(CAN1_EMParasLoss) -> [CAN1_EMParasLoss]
  NFricPercTorq/1(CAN1_NFricPercTorq) -> [CAN1_NFricPercTorq]
  bus_selector/1 -> EMParasLoss/1(EMParasLoss)  "<VOUTP_EEC3EMPressLoss_pct>"
  [BOUTP_outputs] -> bus_selector/1
  bus_selector1/1 -> NFricPercTorq/1(NFricPercTorq)  "<VOUTP_EEC3NFricPercTorq_pct>"
  [BOUTP_outputs] -> bus_selector1/1

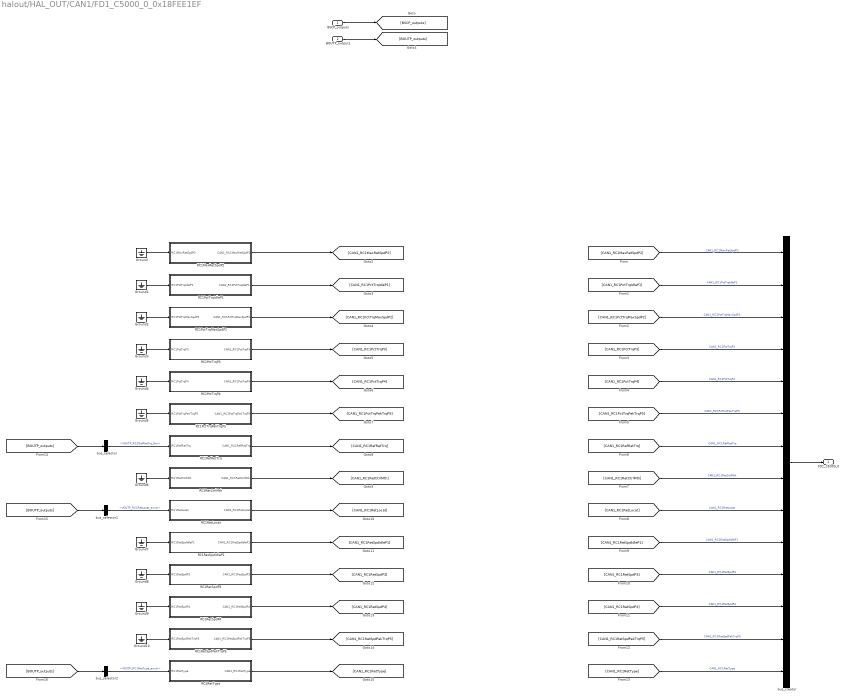
== system halout/HAL_OUT/CAN1/FD1_C5000_0_0x18FEE1EF ==
  BSCP_outputs : Inport  OutDataTypeStr=Bus: BSCP_outputs
  BOUTP_outputs : Inport  Port=2  OutDataTypeStr=Bus: BOUTP_outputs
  Ground{,1..10} (11 alike) : Ground
  RC1MaxRetSpdP2 : Subsystem
  RC1PctTrqIdleP1 : Subsystem
  RC1PctTrqMaxSpdP2 : Subsystem
  RC1PctTrqP3 : Subsystem
  RC1PctTrqP4 : Subsystem
  RC1PctTrqPekTrqP5 : Subsystem
  RC1RefRetTrq : Subsystem
  RC1RetCtrlMth : Subsystem
  RC1RetLocat : Subsystem
  RC1RetSpdIdleP1 : Subsystem
  RC1RetSpdP3 : Subsystem
  RC1RetSpdP4 : Subsystem
  RC1RetSpdPekTrqP5 : Subsystem
  RC1RetType : Subsystem
  bus_creator : BusCreator  Inputs=14  OutDataTypeStr=Bus: DT_CAN1_SG_FD1_C5000_0  NonVirtualBus=on
  bus_selector : BusSelector  OutputSignals=VOUTP_RC1RefRetTrq_Nm
  bus_selector1 : BusSelector  OutputSignals=VOUTP_RC1RetLocat_enum
  bus_selector2 : BusSelector  OutputSignals=VOUTP_RC1RetType_enum
  FD1_C5000_0 : Outport
  wires:
  BSCP_outputs/1 -> [BSCP_outputs]
  BOUTP_outputs/1 -> [BOUTP_outputs]
  [CAN1_RC1MaxRetSpdP2] -> bus_creator/1  "CAN1_RC1MaxRetSpdP2"
  [CAN1_RC1PctTrqIdleP1] -> bus_creator/2  "CAN1_RC1PctTrqIdleP1"
  [CAN1_RC1PctTrqMaxSpdP2] -> bus_creator/3  "CAN1_RC1PctTrqMaxSpdP2"
  [CAN1_RC1PctTrqP3] -> bus_creator/4  "CAN1_RC1PctTrqP3"
  [CAN1_RC1PctTrqP4] -> bus_creator/5  "CAN1_RC1PctTrqP4"
  [CAN1_RC1PctTrqPekTrqP5] -> bus_creator/6  "CAN1_RC1PctTrqPekTrqP5"
  [CAN1_RC1RefRetTrq] -> bus_creator/7  "CAN1_RC1RefRetTrq"
  [CAN1_RC1RetCtrlMth] -> bus_creator/8  "CAN1_RC1RetCtrlMth"
  [CAN1_RC1RetLocat] -> bus_creator/9  "CAN1_RC1RetLocat"
  [CAN1_RC1RetSpdIdleP1] -> bus_creator/10  "CAN1_RC1RetSpdIdleP1"
  [CAN1_RC1RetSpdP3] -> bus_creator/11  "CAN1_RC1RetSpdP3"
  [CAN1_RC1RetSpdP4] -> bus_creator/12  "CAN1_RC1RetSpdP4"
  [CAN1_RC1RetSpdPekTrqP5] -> bus_creator/13  "CAN1_RC1RetSpdPekTrqP5"
  [CAN1_RC1RetType] -> bus_creator/14  "CAN1_RC1RetType"
  bus_creator/1 -> FD1_C5000_0/1
  RC1MaxRetSpdP2/1(CAN1_RC1MaxRetSpdP2) -> [CAN1_RC1MaxRetSpdP2]
  RC1PctTrqIdleP1/1(CAN1_RC1PctTrqIdleP1) -> [CAN1_RC1PctTrqIdleP1]
  RC1PctTrqMaxSpdP2/1(CAN1_RC1PctTrqMaxSpdP2) -> [CAN1_RC1PctTrqMaxSpdP2]
  RC1PctTrqP3/1(CAN1_RC1PctTrqP3) -> [CAN1_RC1PctTrqP3]
  RC1PctTrqP4/1(CAN1_RC1PctTrqP4) -> [CAN1_RC1PctTrqP4]
  RC1PctTrqPekTrqP5/1(CAN1_RC1PctTrqPekTrqP5) -> [CAN1_RC1PctTrqPekTrqP5]
  RC1RefRetTrq/1(CAN1_RC1RefRetTrq) -> [CAN1_RC1RefRetTrq]
  RC1RetCtrlMth/1(CAN1_RC1RetCtrlMth) -> [CAN1_RC1RetCtrlMth]
  RC1RetLocat/1(CAN1_RC1RetLocat) -> [CAN1_RC1RetLocat]
  RC1RetSpdIdleP1/1(CAN1_RC1RetSpdIdleP1) -> [CAN1_RC1RetSpdIdleP1]
  RC1RetSpdP3/1(CAN1_RC1RetSpdP3) -> [CAN1_RC1RetSpdP3]
  RC1RetSpdP4/1(CAN1_RC1RetSpdP4) -> [CAN1_RC1RetSpdP4]
  RC1RetSpdPekTrqP5/1(CAN1_RC1RetSpdPekTrqP5) -> [CAN1_RC1RetSpdPekTrqP5]
  RC1RetType/1(CAN1_RC1RetType) -> [CAN1_RC1RetType]
  Ground/1 -> RC1MaxRetSpdP2/1(RC1MaxRetSpdP2)
  Ground1/1 -> RC1PctTrqIdleP1/1(RC1PctTrqIdleP1)
  Ground2/1 -> RC1PctTrqMaxSpdP2/1(RC1PctTrqMaxSpdP2)
  Ground3/1 -> RC1PctTrqP3/1(RC1PctTrqP3)
  Ground4/1 -> RC1PctTrqP4/1(RC1PctTrqP4)
  Ground5/1 -> RC1PctTrqPekTrqP5/1(RC1PctTrqPekTrqP5)
  bus_selector/1 -> RC1RefRetTrq/1(RC1RefRetTrq)  "<VOUTP_RC1RefRetTrq_Nm>"
  [BOUTP_outputs] -> bus_selector/1
  Ground6/1 -> RC1RetCtrlMth/1(RC1RetCtrlMth)
  bus_selector1/1 -> RC1RetLocat/1(RC1RetLocat)  "<VOUTP_RC1RetLocat_enum>"
  [BOUTP_outputs] -> bus_selector1/1
  Ground7/1 -> RC1RetSpdIdleP1/1(RC1RetSpdIdleP1)
  Ground8/1 -> RC1RetSpdP3/1(RC1RetSpdP3)
  Ground9/1 -> RC1RetSpdP4/1(RC1RetSpdP4)
  Ground10/1 -> RC1RetSpdPekTrqP5/1(RC1RetSpdPekTrqP5)
  bus_selector2/1 -> RC1RetType/1(RC1RetType)  "<VOUTP_RC1RetType_enum>"
  [BOUTP_outputs] -> bus_selector2/1

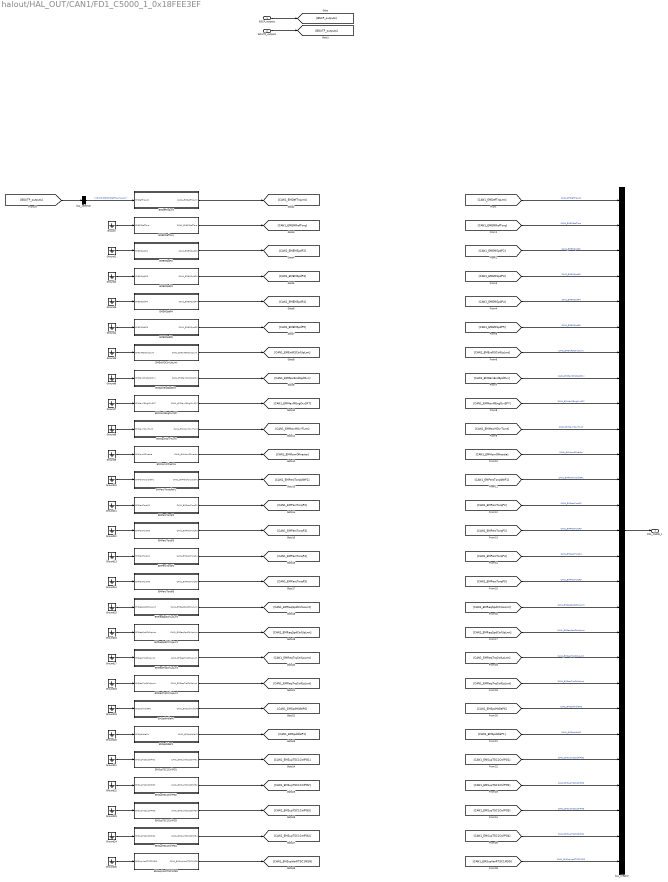
== system halout/HAL_OUT/CAN1/FD1_C5000_1_0x18FEE3EF ==
  BSCP_outputs : Inport  OutDataTypeStr=Bus: BSCP_outputs
  BOUTP_outputs : Inport  Port=2  OutDataTypeStr=Bus: BOUTP_outputs
  EMDefTrqLmt : Subsystem
  EMEMRefTorq : Subsystem
  EMEMSpdP2 : Subsystem
  EMEMSpdP3 : Subsystem
  EMEMSpdP4 : Subsystem
  EMEMSpdP5 : Subsystem
  EMExtRSCtrlUpLmt : Subsystem
  EMGainEndSpdGvn : Subsystem
  EMMaxMEngOvrSP7 : Subsystem
  EMMaxMOvrTLmt : Subsystem
  EMMomOfInertia : Subsystem
  EMPercTorqIdleP1 : Subsystem
  EMPercTorqP2 : Subsystem
  EMPercTorqP3 : Subsystem
  EMPercTorqP4 : Subsystem
  EMPercTorqP5 : Subsystem
  EMReqSpdCtrlLoLmt : Subsystem
  EMReqSpdCtrlUpLmt : Subsystem
  EMReqTrqCtrlLoLmt : Subsystem
  EMReqTrqCtrlUpLmt : Subsystem
  EMSpdHIdleP6 : Subsystem
  EMSpdIdleP1 : Subsystem
  EMSupTSC1CtrlPG1 : Subsystem
  EMSupTSC1CtrlPG2 : Subsystem
  EMSupTSC1CtrlPG3 : Subsystem
  EMSupTSC1CtrlPG4 : Subsystem
  EMSupVarRTSC1MSG : Subsystem
  Ground{,1..25} (26 alike) : Ground
  bus_creator : BusCreator  Inputs=27  OutDataTypeStr=Bus: DT_CAN1_SG_FD1_C5000_1  NonVirtualBus=on
  bus_selector : BusSelector  OutputSignals=VOUTP_EC1EMDefTrqLmt_rpm
  FD1_C5000_1 : Outport
  wires:
  BSCP_outputs/1 -> [BSCP_outputs]
  BOUTP_outputs/1 -> [BOUTP_outputs]
  [CAN1_EMDefTrqLmt] -> bus_creator/1  "CAN1_EMDefTrqLmt"
  [CAN1_EMEMRefTorq] -> bus_creator/2  "CAN1_EMEMRefTorq"
  [CAN1_EMEMSpdP2] -> bus_creator/3  "CAN1_EMEMSpdP2"
  [CAN1_EMEMSpdP3] -> bus_creator/4  "CAN1_EMEMSpdP3"
  [CAN1_EMEMSpdP4] -> bus_creator/5  "CAN1_EMEMSpdP4"
  [CAN1_EMEMSpdP5] -> bus_creator/6  "CAN1_EMEMSpdP5"
  [CAN1_EMExtRSCtrlUpLmt] -> bus_creator/7  "CAN1_EMExtRSCtrlUpLmt"
  [CAN1_EMGainEndSpdGvn] -> bus_creator/8  "CAN1_EMGainEndSpdGvn"
  [CAN1_EMMaxMEngOvrSP7] -> bus_creator/9  "CAN1_EMMaxMEngOvrSP7"
  [CAN1_EMMaxMOvrTLmt] -> bus_creator/10  "CAN1_EMMaxMOvrTLmt"
  [CAN1_EMMomOfInertia] -> bus_creator/11  "CAN1_EMMomOfInertia"
  [CAN1_EMPercTorqIdleP1] -> bus_creator/12  "CAN1_EMPercTorqIdleP1"
  [CAN1_EMPercTorqP2] -> bus_creator/13  "CAN1_EMPercTorqP2"
  [CAN1_EMPercTorqP3] -> bus_creator/14  "CAN1_EMPercTorqP3"
  [CAN1_EMPercTorqP4] -> bus_creator/15  "CAN1_EMPercTorqP4"
  [CAN1_EMPercTorqP5] -> bus_creator/16  "CAN1_EMPercTorqP5"
  [CAN1_EMReqSpdCtrlLoLmt] -> bus_creator/17  "CAN1_EMReqSpdCtrlLoLmt"
  [CAN1_EMReqSpdCtrlUpLmt] -> bus_creator/18  "CAN1_EMReqSpdCtrlUpLmt"
  [CAN1_EMReqTrqCtrlLoLmt] -> bus_creator/19  "CAN1_EMReqTrqCtrlLoLmt"
  [CAN1_EMReqTrqCtrlUpLmt] -> bus_creator/20  "CAN1_EMReqTrqCtrlUpLmt"
  [CAN1_EMSpdHIdleP6] -> bus_creator/21  "CAN1_EMSpdHIdleP6"
  [CAN1_EMSpdIdleP1] -> bus_creator/22  "CAN1_EMSpdIdleP1"
  [CAN1_EMSupTSC1CtrlPG1] -> bus_creator/23  "CAN1_EMSupTSC1CtrlPG1"
  [CAN1_EMSupTSC1CtrlPG2] -> bus_creator/24  "CAN1_EMSupTSC1CtrlPG2"
  [CAN1_EMSupTSC1CtrlPG3] -> bus_creator/25  "CAN1_EMSupTSC1CtrlPG3"
  [CAN1_EMSupTSC1CtrlPG4] -> bus_creator/26  "CAN1_EMSupTSC1CtrlPG4"
  [CAN1_EMSupVarRTSC1MSG] -> bus_creator/27  "CAN1_EMSupVarRTSC1MSG"
  bus_creator/1 -> FD1_C5000_1/1
  EMDefTrqLmt/1(CAN1_EMDefTrqLmt) -> [CAN1_EMDefTrqLmt]
  EMEMRefTorq/1(CAN1_EMEMRefTorq) -> [CAN1_EMEMRefTorq]
  EMEMSpdP2/1(CAN1_EMEMSpdP2) -> [CAN1_EMEMSpdP2]
  EMEMSpdP3/1(CAN1_EMEMSpdP3) -> [CAN1_EMEMSpdP3]
  EMEMSpdP4/1(CAN1_EMEMSpdP4) -> [CAN1_EMEMSpdP4]
  EMEMSpdP5/1(CAN1_EMEMSpdP5) -> [CAN1_EMEMSpdP5]
  EMExtRSCtrlUpLmt/1(CAN1_EMExtRSCtrlUpLmt) -> [CAN1_EMExtRSCtrlUpLmt]
  EMGainEndSpdGvn/1(CAN1_EMGainEndSpdGvn) -> [CAN1_EMGainEndSpdGvn]
  EMMaxMEngOvrSP7/1(CAN1_EMMaxMEngOvrSP7) -> [CAN1_EMMaxMEngOvrSP7]
  EMMaxMOvrTLmt/1(CAN1_EMMaxMOvrTLmt) -> [CAN1_EMMaxMOvrTLmt]
  EMMomOfInertia/1(CAN1_EMMomOfInertia) -> [CAN1_EMMomOfInertia]
  EMPercTorqIdleP1/1(CAN1_EMPercTorqIdleP1) -> [CAN1_EMPercTorqIdleP1]
  EMPercTorqP2/1(CAN1_EMPercTorqP2) -> [CAN1_EMPercTorqP2]
  EMPercTorqP3/1(CAN1_EMPercTorqP3) -> [CAN1_EMPercTorqP3]
  EMPercTorqP4/1(CAN1_EMPercTorqP4) -> [CAN1_EMPercTorqP4]
  EMPercTorqP5/1(CAN1_EMPercTorqP5) -> [CAN1_EMPercTorqP5]
  EMReqSpdCtrlLoLmt/1(CAN1_EMReqSpdCtrlLoLmt) -> [CAN1_EMReqSpdCtrlLoLmt]
  EMReqSpdCtrlUpLmt/1(CAN1_EMReqSpdCtrlUpLmt) -> [CAN1_EMReqSpdCtrlUpLmt]
  EMReqTrqCtrlLoLmt/1(CAN1_EMReqTrqCtrlLoLmt) -> [CAN1_EMReqTrqCtrlLoLmt]
  EMReqTrqCtrlUpLmt/1(CAN1_EMReqTrqCtrlUpLmt) -> [CAN1_EMReqTrqCtrlUpLmt]
  EMSpdHIdleP6/1(CAN1_EMSpdHIdleP6) -> [CAN1_EMSpdHIdleP6]
  EMSpdIdleP1/1(CAN1_EMSpdIdleP1) -> [CAN1_EMSpdIdleP1]
  EMSupTSC1CtrlPG1/1(CAN1_EMSupTSC1CtrlPG1) -> [CAN1_EMSupTSC1CtrlPG1]
  EMSupTSC1CtrlPG2/1(CAN1_EMSupTSC1CtrlPG2) -> [CAN1_EMSupTSC1CtrlPG2]
  EMSupTSC1CtrlPG3/1(CAN1_EMSupTSC1CtrlPG3) -> [CAN1_EMSupTSC1CtrlPG3]
  EMSupTSC1CtrlPG4/1(CAN1_EMSupTSC1CtrlPG4) -> [CAN1_EMSupTSC1CtrlPG4]
  EMSupVarRTSC1MSG/1(CAN1_EMSupVarRTSC1MSG) -> [CAN1_EMSupVarRTSC1MSG]
  bus_selector/1 -> EMDefTrqLmt/1(EMDefTrqLmt)  "<VOUTP_EC1EMDefTrqLmt_rpm>"
  [BOUTP_outputs] -> bus_selector/1
  Ground/1 -> EMEMRefTorq/1(EMEMRefTorq)
  Ground1/1 -> EMEMSpdP2/1(EMEMSpdP2)
  Ground2/1 -> EMEMSpdP3/1(EMEMSpdP3)
  Ground3/1 -> EMEMSpdP4/1(EMEMSpdP4)
  Ground4/1 -> EMEMSpdP5/1(EMEMSpdP5)
  Ground5/1 -> EMExtRSCtrlUpLmt/1(EMExtRSCtrlUpLmt)
  Ground6/1 -> EMGainEndSpdGvn/1(EMGainEndSpdGvn)
  Ground7/1 -> EMMaxMEngOvrSP7/1(EMMaxMEngOvrSP7)
  Ground8/1 -> EMMaxMOvrTLmt/1(EMMaxMOvrTLmt)
  Ground9/1 -> EMMomOfInertia/1(EMMomOfInertia)
  Ground10/1 -> EMPercTorqIdleP1/1(EMPercTorqIdleP1)
  Ground11/1 -> EMPercTorqP2/1(EMPercTorqP2)
  Ground12/1 -> EMPercTorqP3/1(EMPercTorqP3)
  Ground13/1 -> EMPercTorqP4/1(EMPercTorqP4)
  Ground14/1 -> EMPercTorqP5/1(EMPercTorqP5)
  Ground15/1 -> EMReqSpdCtrlLoLmt/1(EMReqSpdCtrlLoLmt)
  Ground16/1 -> EMReqSpdCtrlUpLmt/1(EMReqSpdCtrlUpLmt)
  Ground17/1 -> EMReqTrqCtrlLoLmt/1(EMReqTrqCtrlLoLmt)
  Ground18/1 -> EMReqTrqCtrlUpLmt/1(EMReqTrqCtrlUpLmt)
  Ground19/1 -> EMSpdHIdleP6/1(EMSpdHIdleP6)
  Ground20/1 -> EMSpdIdleP1/1(EMSpdIdleP1)
  Ground21/1 -> EMSupTSC1CtrlPG1/1(EMSupTSC1CtrlPG1)
  Ground22/1 -> EMSupTSC1CtrlPG2/1(EMSupTSC1CtrlPG2)
  Ground23/1 -> EMSupTSC1CtrlPG3/1(EMSupTSC1CtrlPG3)
  Ground24/1 -> EMSupTSC1CtrlPG4/1(EMSupTSC1CtrlPG4)
  Ground25/1 -> EMSupVarRTSC1MSG/1(EMSupVarRTSC1MSG)
